simulink model "Phase_5PWM"  (R2017b)
settings: Solver=VariableStepAuto  StartTime=0.0  StopTime=0.4  MaxStep=1e-4  RelTol=1e-3
undefined symbols (not defined in the file): f
libraries: powerlib x25, powerlib_meascontrol x5
settings Model: Creator=admin  LastModifiedBy=admin

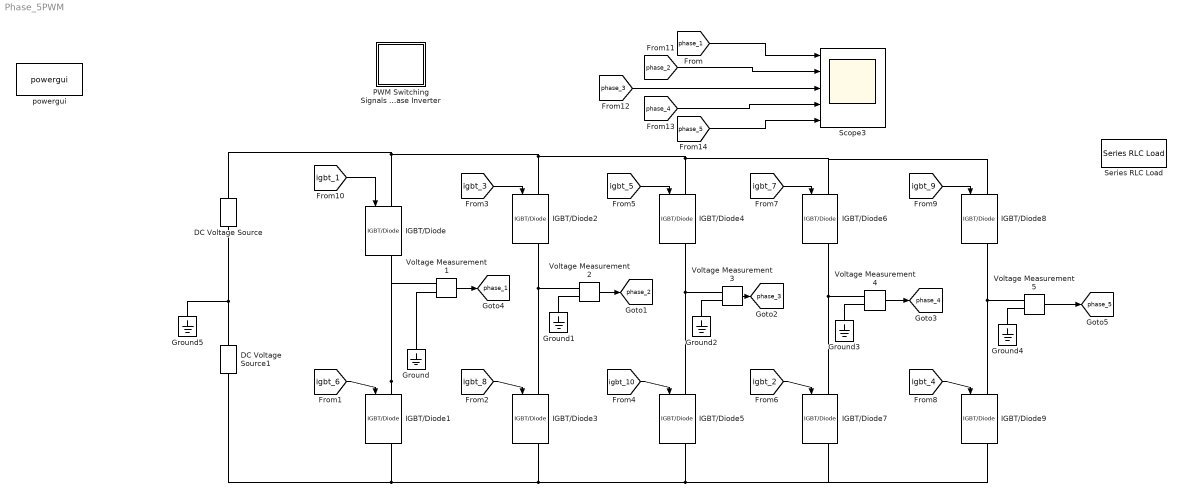
== system Phase_5PWM ==
  DC Voltage Source : powerlib/Electrical Sources/DC Voltage Source  Amplitude=100  Measurements=None
  DC Voltage Source1 : powerlib/Electrical Sources/DC Voltage Source  Amplitude=100  Measurements=None
  Ground{,1..5} (6 alike) : powerlib/Elements/Ground  LConnTagsString=a
  IGBT/Diode{,1..9} (10 alike) : powerlib/Power Electronics/IGBT//Diode  Ron=1e-3  Rs=1e5  Cs=inf  Measurements=on
  "PWM Switching Signals for 5 Phase Inverter " : Subsystem
  Scope3 : Scope  NumInputPorts=5
  Series RLC Load : powerlib/Elements/Series RLC Load  LConnTagsString=a  RConnTagsString=__new0  NominalVoltage=1000  NominalFrequency=60  ActivePower=10e3  InductivePower=100  CapacitivePower=100  Setx0=off  InitialVoltage=0  SetiL0=off  InitialCurrent=0  Measurements=None  LoadType=constant Z
  Voltage Measurement{1..5} (5 alike) : powerlib/Measurements/Voltage Measurement  PhasorSimulation=off  OutputType=Complex  PSBequivalent=0
  powergui : powerlib/powergui  Priority=1  SimulationMode=Continuous  SampleTime=50e-6  frequency=60  Iterations=50  frequencyindice=0  Pbase=100e6  ErrMax=1e-4  UnitsV=kV  UnitsW=MW  buscounter=0  FunctionMessages=off  echomessages=off  EnableUseOfTLC=off  CurrentSourceSwitches=off  DisableSnubberDevices=off  DisableRonSwitches=off  DisableVfSwitches=off  DisplayEquations=off  SolverType=Tustin/Backward Euler (TBE)  Interpol=off  ExternalGateDelay=off  methode=off  Ts=100  x0status=blocks  SPID=on  SwTol=0  HookPort=off  RestoreLinks=warning  ResistiveCurrentMeasurement=off  Frange=[0:2:500]  Ylog=off  Xlog=on  ShowGrid=off  save=off  variable=ZData  structure=0  ZoomFFT=off  StartTime=0.0  cycles=1  DisplayStyle=1  fundamental=60  FreqAxis=off  MaxFrequency=1000  frequencyindicesteady=1  RmsSteady=1  display=off
  tag scope: phase_1=global, phase_2=global, phase_3=global, phase_4=global, phase_5=global
  wires:
  [phase_1] -> Scope3/1
  [igbt_6] -> IGBT/Diode1/1
  Voltage Measurement3/1 -> [phase_3]
  [igbt_1] -> IGBT/Diode/1
  [phase_2] -> Scope3/2
  [igbt_7] -> IGBT/Diode6/1
  [igbt_8] -> IGBT/Diode3/1
  [igbt_2] -> IGBT/Diode7/1
  Voltage Measurement5/1 -> [phase_5]
  [igbt_10] -> IGBT/Diode5/1
  [phase_4] -> Scope3/4
  [igbt_4] -> IGBT/Diode9/1
  Voltage Measurement1/1 -> [phase_1]
  [igbt_3] -> IGBT/Diode2/1
  [phase_5] -> Scope3/5
  [igbt_5] -> IGBT/Diode4/1
  Voltage Measurement2/1 -> [phase_2]
  [phase_3] -> Scope3/3
  [igbt_9] -> IGBT/Diode8/1
  Voltage Measurement4/1 -> [phase_4]
  connections:
  IGBT/Diode4/RConn1 -- Voltage Measurement3/LConn1 -- IGBT/Diode5/LConn1
  IGBT/Diode3/RConn1 -- IGBT/Diode9/RConn1 -- IGBT/Diode7/RConn1 -- IGBT/Diode5/RConn1 -- DC Voltage Source1/LConn1 -- IGBT/Diode1/RConn1
  IGBT/Diode1/LConn1 -- IGBT/Diode/RConn1 -- Voltage Measurement1/LConn1
  IGBT/Diode6/RConn1 -- Voltage Measurement4/LConn1 -- IGBT/Diode7/LConn1
  IGBT/Diode4/LConn1 -- IGBT/Diode8/LConn1 -- IGBT/Diode6/LConn1 -- IGBT/Diode/LConn1 -- DC Voltage Source/RConn1 -- IGBT/Diode2/LConn1
  DC Voltage Source1/RConn1 -- Ground5/LConn1 -- DC Voltage Source/LConn1
  IGBT/Diode8/RConn1 -- Voltage Measurement5/LConn1 -- IGBT/Diode9/LConn1
  IGBT/Diode2/RConn1 -- Voltage Measurement2/LConn1 -- IGBT/Diode3/LConn1
  Voltage Measurement4/LConn2 -- Ground3/LConn1
  Voltage Measurement5/LConn2 -- Ground4/LConn1
  Voltage Measurement3/LConn2 -- Ground2/LConn1
  Voltage Measurement1/LConn2 -- Ground/LConn1
  Voltage Measurement2/LConn2 -- Ground1/LConn1

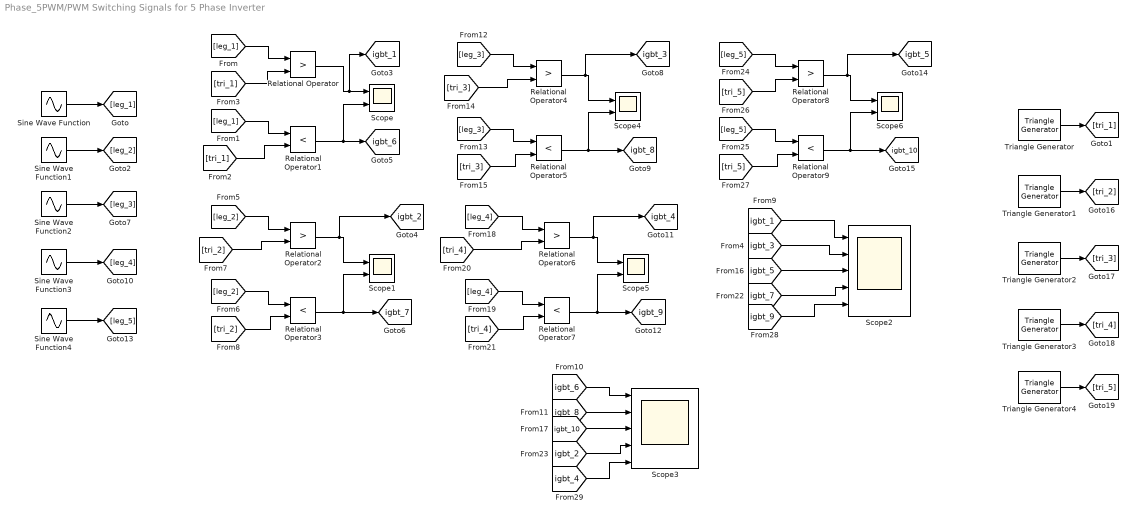
== system Phase_5PWM/PWM Switching Signals for 5 Phase Inverter  ==
  Relational Operator{,2,4,6,8} (5 alike) : RelationalOperator  Operator=>  OutDataTypeStr=boolean  RndMeth=Simplest
  Relational Operator{1,3,5,7,9} (5 alike) : RelationalOperator  Operator=<  OutDataTypeStr=boolean  RndMeth=Simplest
  Scope{,1,4..6} (5 alike) : Scope  NumInputPorts=2
  Scope2 : Scope  NumInputPorts=5
  Scope3 : Scope  NumInputPorts=5
  Sine Wave Function : Sin  Frequency=2*pi*f  SampleTime=0
  Sine Wave Function1 : Sin  Frequency=2*pi*f  Phase=-pi/5  SampleTime=0
  Sine Wave Function2 : Sin  Frequency=2*pi*f  Phase=-(2*pi)/5  SampleTime=0
  Sine Wave Function3 : Sin  Frequency=2*pi*f  Phase=-(3*pi)/5  SampleTime=0
  Sine Wave Function4 : Sin  Frequency=2*pi*f  Phase=-(4*pi)/5  SampleTime=0
  Triangle Generator : powerlib_meascontrol/Pulse & Signal Generators/Triangle Generator  Freq=2*pi*f*10  Phase=0  Ts=0
  Triangle Generator1 : powerlib_meascontrol/Pulse & Signal Generators/Triangle Generator  Freq=2*pi*f*10  Phase=-180/5  Ts=0
  Triangle Generator2 : powerlib_meascontrol/Pulse & Signal Generators/Triangle Generator  Freq=2*pi*f*10  Phase=-2*180/5  Ts=0
  Triangle Generator3 : powerlib_meascontrol/Pulse & Signal Generators/Triangle Generator  Freq=2*pi*f*10  Phase=-3*180/5  Ts=0
  Triangle Generator4 : powerlib_meascontrol/Pulse & Signal Generators/Triangle Generator  Freq=2*pi*f*10  Phase=-4*180/5  Ts=0
  tag scope: igbt_10=global, igbt_1=global, igbt_2=global, igbt_3=global, igbt_4=global, igbt_5=global, igbt_6=global, igbt_7=global, igbt_8=global, igbt_9=global
  wires:
  Sine Wave Function/1 -> [leg_1]
  [tri_1] -> Relational Operator1/2
  [leg_1] -> Relational Operator1/1
  Relational Operator3/1 -> [igbt_7], Scope1/2
  [leg_2] -> Relational Operator2/1
  Relational Operator2/1 -> [igbt_2], Scope1/1
  [tri_2] -> Relational Operator3/2
  [leg_2] -> Relational Operator3/1
  [leg_1] -> Relational Operator/1
  [tri_1] -> Relational Operator/2
  Relational Operator1/1 -> [igbt_6], Scope/2
  Relational Operator/1 -> [igbt_1], Scope/1
  [tri_4] -> Relational Operator6/2
  Sine Wave Function3/1 -> [leg_4]
  [leg_4] -> Relational Operator6/1
  Relational Operator6/1 -> [igbt_4], Scope5/1
  [leg_4] -> Relational Operator7/1
  [tri_4] -> Relational Operator7/2
  Relational Operator7/1 -> [igbt_9], Scope5/2
  [igbt_8] -> Scope3/2
  [igbt_1] -> Scope2/1
  [igbt_6] -> Scope3/1
  [igbt_3] -> Scope2/2
  [igbt_7] -> Scope2/4
  Sine Wave Function1/1 -> [leg_2]
  [leg_5] -> Relational Operator8/1
  [tri_5] -> Relational Operator9/2
  [tri_5] -> Relational Operator8/2
  Relational Operator9/1 -> Scope6/2, [igbt_10]
  Sine Wave Function4/1 -> [leg_5]
  Relational Operator8/1 -> Scope6/1, [igbt_5]
  [leg_5] -> Relational Operator9/1
  [igbt_5] -> Scope2/3
  [leg_3] -> Relational Operator5/1
  Relational Operator5/1 -> Scope4/2, [igbt_8]
  [tri_3] -> Relational Operator5/2
  [leg_3] -> Relational Operator4/1
  Sine Wave Function2/1 -> [leg_3]
  Relational Operator4/1 -> Scope4/1, [igbt_3]
  [igbt_4] -> Scope3/5
  [igbt_10] -> Scope3/3
  [igbt_9] -> Scope2/5
  [igbt_2] -> Scope3/4
  Triangle Generator/1 -> [tri_1]
  Triangle Generator1/1 -> [tri_2]
  Triangle Generator2/1 -> [tri_3]
  Triangle Generator3/1 -> [tri_4]
  Triangle Generator4/1 -> [tri_5]
  [tri_2] -> Relational Operator2/2
  [tri_3] -> Relational Operator4/2
